simulink model "qwert1"  (R2018a)
settings: Solver=VariableStepAuto  StartTime=0.0  StopTime=1  RelTol=1e-3
libraries: powerlib x5, simulink x1, powerlib_meascontrol x1
settings Model: Creator=Emre Deniz  LastModifiedBy=Emre Deniz

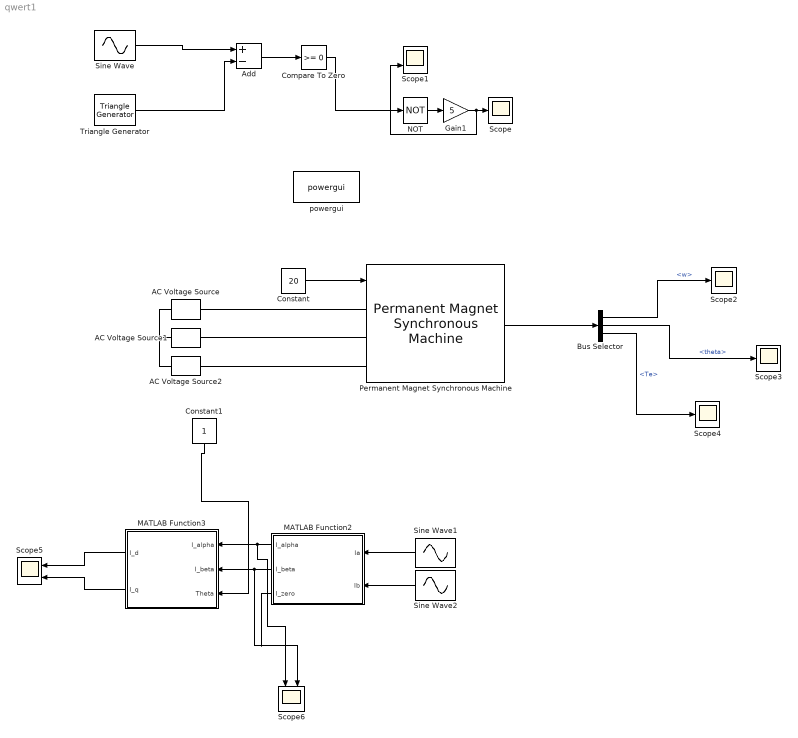
== system qwert1 ==
  AC Voltage Source : powerlib/Electrical Sources/AC Voltage Source  Amplitude=100  Phase=0  Frequency=60  SampleTime=0  Measurements=None  BusType=swing  Pref=10e3  Qref=0  Qmin=-inf  Qmax=+inf
  AC Voltage Source1 : powerlib/Electrical Sources/AC Voltage Source  Amplitude=100  Phase=-120  Frequency=60  SampleTime=0  Measurements=None  BusType=swing  Pref=10e3  Qref=0  Qmin=-inf  Qmax=+inf
  AC Voltage Source2 : powerlib/Electrical Sources/AC Voltage Source  Amplitude=100  Phase=120  Frequency=60  SampleTime=0  Measurements=None  BusType=swing  Pref=10e3  Qref=0  Qmin=-inf  Qmax=+inf
  Add : Sum  Inputs=+-
  Bus Selector : BusSelector  OutputSignals=w,theta,Te
  Compare To Zero : simulink/Logic and Bit Operations/Compare To Zero  relop=>=  OutDataTypeStr=boolean
  Constant : Constant  Value=20
  Constant1 : Constant
  Gain1 : Gain  Gain=5
  MATLAB Function2 : MATLAB Function  TreatAsAtomicUnit=on
  MATLAB Function3 : MATLAB Function  TreatAsAtomicUnit=on
  NOT : Logic  Operator=NOT  IconShape=distinctive  AllPortsSameDT=off  OutDataTypeStr=boolean
  Permanent Magnet Synchronous Machine : powerlib/Machines/Permanent Magnet Synchronous Machine  NbPhases=3  FluxDistribution=Sinusoidal  RotorType=Round  MechanicalLoad=Torque Tm  PresetModel=No  ShowDetailedParameters=on  MeasurementBus=on  Resistance=0.0485  Inductance=8.5e-3  dqInductances=[8.5e-3,8.5e-3]  La=0.000395  MachineConstant=Flux linkage established by magnets (V.s)  Flux=0.1194  VoltageCst=86.6271  TorqueCst=0.7164  Flat=120  Mechanical=[0.0027 0.0004924 4 0]  PolePairs=4  InitialConditions=[30,0, 0,0]  InitialConditions5ph=[0 0 0 0 0 0]  TsPowergui=0  TsBlock=-1  RefAngle=Aligned with phase A axis (original Park)
      settings: SourceProductName=Simscape Power Systems
  Scope{,2..4} (4 alike) : Scope
  Scope1 : Scope  NumInputPorts=2
  Scope5 : Scope  NumInputPorts=2
  Scope6 : Scope  NumInputPorts=2
  Sine Wave : Sin  Frequency=50  SampleTime=0
  Sine Wave1 : Sin  Frequency=50  SampleTime=0
  Sine Wave2 : Sin  Frequency=50  Phase=2*pi/3  SampleTime=0
  Triangle Generator : powerlib_meascontrol/Pulse & Signal Generators/Triangle Generator  Freq=75*21  Phase=90  Ts=0
  powergui : powerlib/powergui  Priority=1  SimulationMode=Continuous  SampleTime=50e-6  frequency=60  Iterations=50  frequencyindice=60  Pbase=100e6  ErrMax=1e-4  UnitsV=kV  UnitsW=MW  buscounter=0  FunctionMessages=off  echomessages=off  EnableUseOfTLC=off  CurrentSourceSwitches=off  DisableSnubberDevices=off  DisableRonSwitches=off  DisableVfSwitches=off  DisplayEquations=off  SolverType=Tustin/Backward Euler (TBE)  Interpol=off  ExternalGateDelay=off  methode=off  Ts=100  x0status=blocks  SPID=on  SwTol=0  HookPort=off  RestoreLinks=warning  ResistiveCurrentMeasurement=off  Frange=[0:2:500]  Ylog=off  Xlog=on  ShowGrid=off  save=off  variable=ZData  structure=0  ZoomFFT=off  StartTime=0.0  cycles=1  DisplayStyle=1  fundamental=60  FreqAxis=off  MaxFrequency=1000  frequencyindicesteady=1  RmsSteady=1  display=off
  wires:
  Add/1 -> Compare To Zero/1
  Triangle Generator/1 -> Add/2
  Sine Wave/1 -> Add/1
  Compare To Zero/1 -> NOT/1
  NOT/1 -> Gain1/1
  Gain1/1 -> Scope1/2, Scope/1
  Constant/1 -> Permanent Magnet Synchronous Machine/1
  Permanent Magnet Synchronous Machine/1 -> Bus Selector/1
  Bus Selector/1 -> Scope2/1  "<w>"
  Bus Selector/2 -> Scope3/1  "<theta>"
  Bus Selector/3 -> Scope4/1  "<Te>"
  MATLAB Function2/3(I_zero) -> ?
  MATLAB Function2/2(I_beta) -> Scope6/2, MATLAB Function3/2(I_beta)
  MATLAB Function2/1(I_alpha) -> Scope6/1, MATLAB Function3/1(I_alpha)
  Constant1/1 -> MATLAB Function3/3(Theta)
  Sine Wave1/1 -> MATLAB Function2/1(Ia)
  Sine Wave2/1 -> MATLAB Function2/2(Ib)
  MATLAB Function3/1(I_d) -> Scope5/1
  MATLAB Function3/2(I_q) -> Scope5/2
  connections:
  Permanent Magnet Synchronous Machine/LConn1 -- AC Voltage Source/RConn1
  AC Voltage Source2/RConn1 -- Permanent Magnet Synchronous Machine/LConn3
  AC Voltage Source1/RConn1 -- Permanent Magnet Synchronous Machine/LConn2
  AC Voltage Source/LConn1 -- AC Voltage Source2/LConn1 -- AC Voltage Source1/LConn1

== matlab function qwert1/MATLAB Function2 ==
  data: Ia input; I_alpha output; Ib input; I_beta output; I_zero output
function [I_alpha, I_beta, I_zero] = Clarke(Ia,Ib)

Ic = - Ia - Ib;

A = (2/3)*[1 -1/2 -1/2 ; 0 sqrt(3)/2 -sqrt(3)/2 ; 1/2 1/2 1/2];

I_in = [Ia ; Ib; Ic];

I_out = A*I_in;

I_alpha = I_out(1);
I_beta = I_out(2);
I_zero = I_out(3);

== matlab function qwert1/MATLAB Function3 ==
  data: I_alpha input; I_d output; I_beta input; I_q output; Theta input
function [I_d, I_q] = Park(I_alpha,I_beta,Theta)

I_in = [I_alpha ; I_beta];

A = [cos(Theta) -sin(Theta) ; sin(Theta) cos(Theta)];

I_out = A*I_in;

I_d = I_out(1);
I_q = I_out(2);
